simulink model "sf_matrix"  (R2017b)
settings: Solver=ode45  StartTime=0.0  StopTime=1  MaxStep=1  RelTol=1e-3  EnableMultiTasking=on
settings Model: FPTRunName=Active  ExtModeAutoUpdateStatusClock=off  Creator=The MathWorks, Inc.  LastModifiedBy=The MathWorks, Inc.
settings DataIOCC: LimitDataPoints=on  SaveFormat=Array
settings OptimizationCC: BooleanDataType=off  ExpressionDepthLimit=2147483647  InitFltsAndDblsToZero=on  EfficientMapNaN2IntZero=off  LifeSpan=inf
settings DebuggingCC: SaveWithParameterizedLinksMsg=none  UnderspecifiedInitializationDetection=Classic  MergeDetectMultiDrivingBlocksExec=none  SignalResolutionControl=TryResolveAllWithWarning  MultiTaskDSMMsg=warning  MultiTaskCondExecSysMsg=none  FcnCallInpInsideContextMsg=warning  StateNameClashWarn=warning  StrictBusMsg=None  SFUnexpectedBacktrackingDiag=warning  SFNoUnconditionalDefaultTransitionDiag=warning  SFExecutionAtInitializationDiag=none
settings HardwareCC: ProdBitPerPointer=32  ProdBitPerSizeT=32  ProdBitPerPtrDiffT=32  ProdLargestAtomicFloat=None  ProdIntDivRoundTo=Undefined  ProdEndianess=Unspecified  ProdWordSize=32  ProdHWDeviceType=32-bit Generic  TargetUnknown=on
settings ModelReferenceCC: PropagateSignalLabelsOutOfModel=off
settings SFSimCC: SimParseCustomCode=off
settings CodeAppCC: StateflowObjectComments=on
settings GRTTargetCC: TargetFcnLib=ansi_tfl_tmw.mat  TargetLangStandard=C89/C90 (ANSI)  GeneratePreprocessorConditionals=Disable all  CombineOutputUpdateFcns=off  GRTInterface=on
settings ConfigComp: CovMetricSettings=dcmtr  CovHtmlReporting=on  CovSaveCumulativeToWorkspaceVar=on  CovSaveSingleToWorkspaceVar=on  CovExternalEMLEnable=off  CovSFcnEnable=off

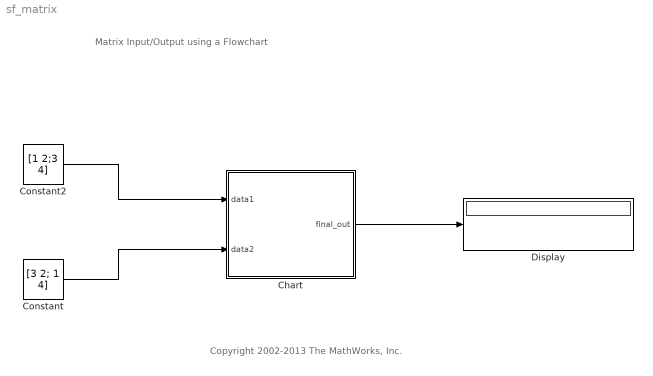
== system sf_matrix ==
  note: Matrix Input/Output using a Flowchart
  note: Copyright 2002-2013 The MathWorks, Inc.
  Chart : Stateflow chart  TreatAsAtomicUnit=on
  Constant : Constant  Value=[3 2; 1 4]  VectorParams1D=off
  Constant2 : Constant  Value=[1 2;3 4]  VectorParams1D=off
  Display : Display
  wires:
  Constant2/1 -> Chart/1(data1)
  Constant/1 -> Chart/2(data2)
  Chart/1(final_out) -> Display/1

== stateflow chart sf_matrix/Chart ==
  note: Equivalent C-Code:
      |
      | for(i=0;i<2;i++)
      |    for(j=0;j<2;j++)
      |        {
      |          int final_out[2][2];
      |          final_out[i][j]=(data1[i][0]*data2[0][j])+(data1[i][1]+data2[1][j]);
      |        }
  (default) -> (junction 7) : {final_out(1,1)=(data1(1,1).*data2(1,1))+(data1(1,2).*data2(2,1));}
  (junction 7) -> (junction 8) : {final_out(1,2)=(data1(1,1).*data2(1,2))+(data1(1,2).*data2(2,2));}
  (junction 8) -> (junction 9) : {final_out(2,1)=(data1(2,1).*data2(1,1))+(data1(2,2).*data2(2,1));}
  (junction 9) -> (junction 10) : {final_out(2,2)=(data1(2,1).*data2(1,2))+(data1(2,2).*data2(2,2));}
  data: final_out output double size=[2 2]; data1 input double size=[2 2]; data2 input double size=[2 2]
